simulink model "Template_TheNotebookEdition"  (R2024b)
settings: Solver=FixedStepAuto  StartTime=0.0  StopTime=inf  RelTol=1e-3  EnableMultiTasking=on
libraries: vexarmcortexlib x24, vexcommonlib x2
settings Model: Creator=ierdn  LastModifiedBy=ierdn
settings DataIOCC: LimitDataPoints=on  SignalLoggingSaveFormat=ModelDataLogs  ReturnWorkspaceOutputs=off
settings OptimizationCC: ExpressionDepthLimit=2147483647  LifeSpan=Inf  MaxStackSize=64  EfficientTunableParamExpr=on
settings DebuggingCC: UnderspecifiedInitializationDetection=Classic  MergeDetectMultiDrivingBlocksExec=none  InheritedTsInSrcMsg=none  FcnCallInpInsideContextMsg=warning  StateNameClashWarn=warning  SFUnexpectedBacktrackingDiag=warning  SFNoUnconditionalDefaultTransitionDiag=warning  SFExecutionAtInitializationDiag=none  ArithmeticOperatorsInVariantConditions=warning
settings HardwareCC: ProdBitPerPointer=32  ProdBitPerSizeT=32  ProdBitPerPtrDiffT=32  ProdLargestAtomicInteger=Long  ProdLargestAtomicFloat=Double  ProdIntDivRoundTo=Undefined  ProdWordSize=32  ProdHWDeviceType=ARM Compatible->ARM Cortex
settings ModelReferenceCC: EnableRefExpFcnMdlSchedulingChecks=on  PropagateSignalLabelsOutOfModel=off
settings SFSimCC: MATLABDynamicMemAlloc=off  CustomCodeUndefinedFunction=UseInterfaceOnly
settings RTWCC: Description=Embedded Coder  SystemTargetFile=ert.tlc  HardwareBoard=ARM Cortex-based VEX Microcontroller  TemplateMakefile=ert_default_tmf  Toolchain=GNU Tools for VEX ARM Cortex  GPUComputeCapability=3.5
settings CodeAppCC: IgnoreCustomStorageClasses=off  CustomSymbolStrType=$N$R$M  StateflowObjectComments=on  InternalIdentifier=Classic
settings ERTTargetCC: CodeReplacementLibrary=GCC ARM Cortex-M3  MultiwordLength=2048  InlinedParameterPlacement=Hierarchical  ConvertIfToSwitch=off  SuppressUnreachableDefaultCases=off  DynamicArrayContainerType=coder::array

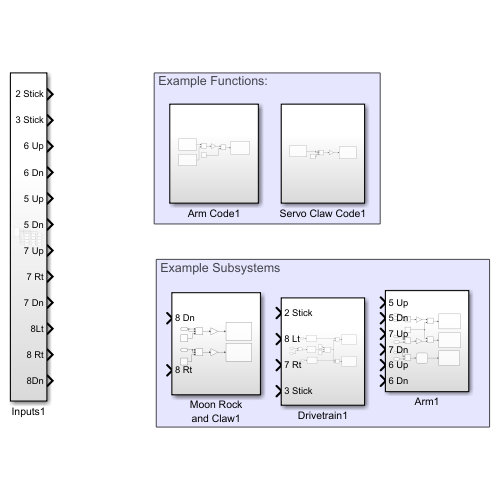
[thumbnail: Simulink's stored preview of the top-level diagram]
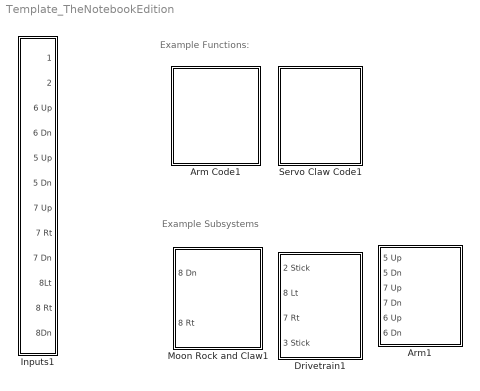
== system Template_TheNotebookEdition ==
  note: Example Functions:
  note: Example Subsystems
  Arm Code1 : Subsystem
  Arm1 : Subsystem
  Drivetrain1 : Subsystem
  Inputs1 : Subsystem
  Moon Rock and Claw1 : Subsystem
  Servo Claw Code1 : Subsystem

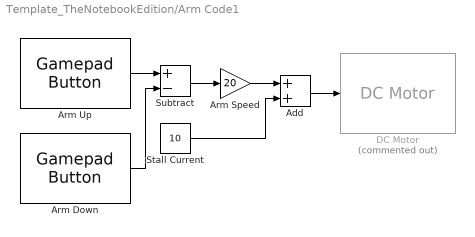
== system Template_TheNotebookEdition/Arm Code1 ==
  Add : Sum
  Arm Down : vexarmcortexlib/Gamepad/Gamepad Button  joystick=1  chan=5  button56=Down  button78=Down  SimulationIn=off  SampleTime=0.02
  Arm Speed : Gain  Gain=20
  Arm Up : vexarmcortexlib/Gamepad/Gamepad Button  joystick=1  chan=5  button56=Up  button78=Down  SimulationIn=off  SampleTime=0.02
  DC Motor : vexarmcortexlib/Actuators/DC Motor  Commented=on  motor=1  scaleFactor=1/13.5  SimulationOut=off
  Stall Current : Constant  Value=10
  Subtract : Sum  Inputs=+-
  wires:
  Arm Speed/1 -> Add/1
  Arm Down/1 -> Subtract/2
  Add/1 -> DC Motor/1
  Stall Current/1 -> Add/2
  Subtract/1 -> Arm Speed/1
  Arm Up/1 -> Subtract/1

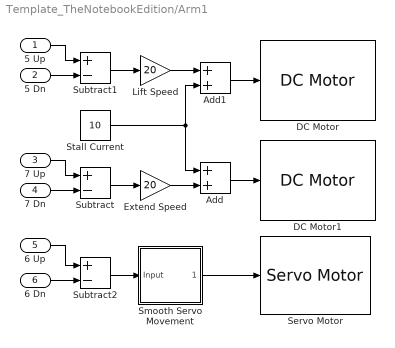
== system Template_TheNotebookEdition/Arm1 ==
  5 Up : Inport
  5 Dn : Inport  Port=2
  7 Up : Inport  Port=3
  7 Dn : Inport  Port=4
  6 Up : Inport  Port=5
  6 Dn : Inport  Port=6
  Add : Sum
  Add1 : Sum
  DC Motor : vexarmcortexlib/Actuators/DC Motor  motor=8  scaleFactor=1/13.5  SimulationOut=off
  DC Motor1 : vexarmcortexlib/Actuators/DC Motor  motor=4  scaleFactor=1/13.5  SimulationOut=off
  Extend Speed : Gain  Gain=20
  Lift Speed : Gain  Gain=20
  Servo Motor : vexarmcortexlib/Actuators/Servo Motor  motor=5  scaleFactor=60/127  SimulationOut=off
  Smooth Servo Movement : Stateflow chart  TreatAsAtomicUnit=on
  Stall Current : Constant  Value=10
  Subtract : Sum  Inputs=+-
  Subtract1 : Sum  Inputs=+-
  Subtract2 : Sum  Inputs=+-
  wires:
  5 Up/1 -> Subtract1/1
  Lift Speed/1 -> Add1/1
  Add1/1 -> DC Motor/1
  Stall Current/1 -> Add/1, Add1/2
  Subtract1/1 -> Lift Speed/1
  5 Dn/1 -> Subtract1/2
  Add/1 -> DC Motor1/1
  7 Dn/1 -> Subtract/2
  Subtract/1 -> Extend Speed/1
  Extend Speed/1 -> Add/2
  7 Up/1 -> Subtract/1
  6 Up/1 -> Subtract2/1
  6 Dn/1 -> Subtract2/2
  Subtract2/1 -> Smooth Servo Movement/1(Input)
  Smooth Servo Movement/1(Output) -> Servo Motor/1

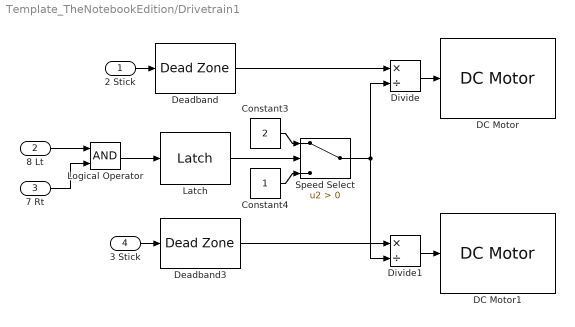
== system Template_TheNotebookEdition/Drivetrain1 ==
  2 Stick : Inport
  8 Lt : Inport  Port=2
  7 Rt : Inport  Port=3
  3 Stick : Inport  Port=4
  Constant3 : Constant  Value=2
  Constant4 : Constant
  DC Motor : vexarmcortexlib/Actuators/DC Motor  motor=2  scaleFactor=1/13.5  SimulationOut=off
  DC Motor1 : vexarmcortexlib/Actuators/DC Motor  motor=9  scaleFactor=1/13.5  SimulationOut=off
  Deadband : DeadZone  LowerValue=-9  UpperValue=9
  Deadband3 : DeadZone  LowerValue=-9  UpperValue=9
  Divide : Product  Inputs=*/
  Divide1 : Product  Inputs=*/
  Latch : vexcommonlib/Latch  output0=off  BlockPlatform=vexarmcortex
  Logical Operator : Logic  AllPortsSameDT=off  OutDataTypeStr=boolean
  Speed Select : Switch  Criteria=u2 > Threshold  SaturateOnIntegerOverflow=off  InputSameDT=off
  wires:
  Speed Select/1 -> Divide/2, Divide1/2
  Latch/1 -> Speed Select/2
  Constant3/1 -> Speed Select/1
  Deadband3/1 -> Divide1/1
  Constant4/1 -> Speed Select/3
  Deadband/1 -> Divide/1
  Divide/1 -> DC Motor/1
  3 Stick/1 -> Deadband3/1
  2 Stick/1 -> Deadband/1
  Divide1/1 -> DC Motor1/1
  8 Lt/1 -> Logical Operator/1
  7 Rt/1 -> Logical Operator/2
  Logical Operator/1 -> Latch/1

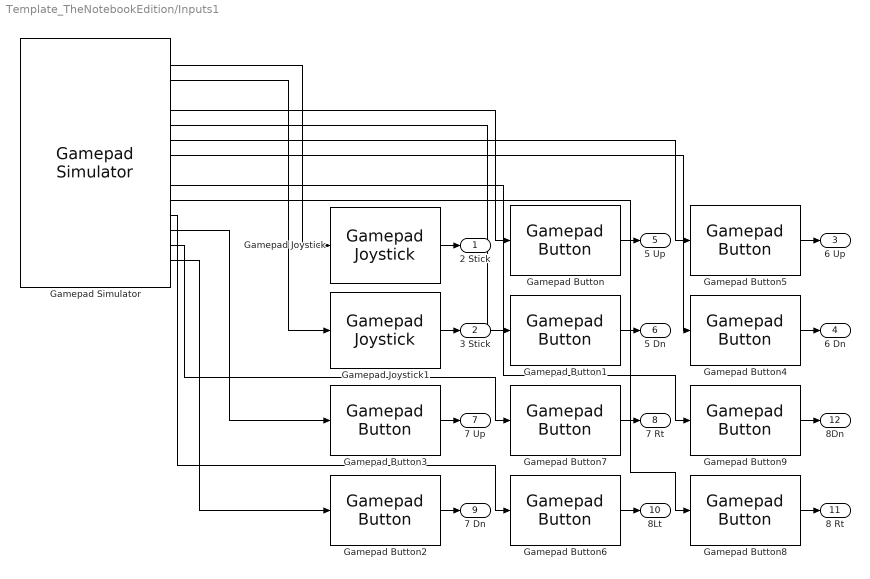
== system Template_TheNotebookEdition/Inputs1 ==
  Gamepad Button : vexarmcortexlib/Gamepad/Gamepad Button  joystick=1  chan=5  button56=Up  button78=Down  SimulationIn=on  SampleTime=0.02
  Gamepad Button1 : vexarmcortexlib/Gamepad/Gamepad Button  joystick=1  chan=5  button56=Down  button78=Down  SimulationIn=on  SampleTime=0.02
  Gamepad Button2 : vexarmcortexlib/Gamepad/Gamepad Button  joystick=1  chan=7  button56=Up  button78=Down  SimulationIn=on  SampleTime=0.02
  Gamepad Button3 : vexarmcortexlib/Gamepad/Gamepad Button  joystick=1  chan=7  button56=Up  button78=Up  SimulationIn=on  SampleTime=0.02
  Gamepad Button4 : vexarmcortexlib/Gamepad/Gamepad Button  joystick=1  chan=6  button56=Down  button78=Down  SimulationIn=on  SampleTime=0.02
  Gamepad Button5 : vexarmcortexlib/Gamepad/Gamepad Button  joystick=1  chan=6  button56=Up  button78=Down  SimulationIn=on  SampleTime=0.02
  Gamepad Button6 : vexarmcortexlib/Gamepad/Gamepad Button  joystick=1  chan=8  button56=Up  button78=Left  SimulationIn=on  SampleTime=0.02
  Gamepad Button7 : vexarmcortexlib/Gamepad/Gamepad Button  joystick=1  chan=7  button56=Up  button78=Right  SimulationIn=on  SampleTime=0.02
  Gamepad Button8 : vexarmcortexlib/Gamepad/Gamepad Button  joystick=1  chan=8  button56=Up  button78=Right  SimulationIn=on  SampleTime=0.02
  Gamepad Button9 : vexarmcortexlib/Gamepad/Gamepad Button  joystick=1  chan=8  button56=Up  button78=Down  SimulationIn=on  SampleTime=0.02
  Gamepad Joystick : vexarmcortexlib/Gamepad/Gamepad Joystick  joystick=1  chan=2  SimulationIn=on  SampleTime=0.02
  Gamepad Joystick1 : vexarmcortexlib/Gamepad/Gamepad Joystick  joystick=1  chan=3  SimulationIn=on  SampleTime=0.02
  Gamepad Simulator : vexcommonlib/Gamepad Simulator  WhichPad=Logitech Gamepad  JoyId=1  BlockPlatform=vexarmcortex
      settings: LibrarySourceBlock=vexarmcortexlib/Utilities/Gamepad Simulator
  " 2 Stick" : Outport
  3 Stick : Outport  Port=2
  6 Up : Outport  Port=3
  6 Dn : Outport  Port=4
  5 Up : Outport  Port=5
  5 Dn : Outport  Port=6
  7 Up : Outport  Port=7
  7 Rt : Outport  Port=8
  7 Dn : Outport  Port=9
  8Lt : Outport  Port=10
  8 Rt : Outport  Port=11
  8Dn : Outport  Port=12
  wires:
  Gamepad Button5/1 -> 6 Up/1
  Gamepad Joystick1/1 -> 3 Stick/1
  Gamepad Button9/1 -> 8Dn/1
  Gamepad Button6/1 -> 8Lt/1
  Gamepad Button7/1 -> 7 Rt/1
  Gamepad Button4/1 -> 6 Dn/1
  Gamepad Button1/1 -> 5 Dn/1
  Gamepad Button/1 -> 5 Up/1
  Gamepad Button8/1 -> 8 Rt/1
  Gamepad Button3/1 -> 7 Up/1
  Gamepad Button2/1 -> 7 Dn/1
  Gamepad Joystick/1 -> " 2 Stick"/1
  Gamepad Simulator/2 -> Gamepad Joystick/1
  Gamepad Simulator/3 -> Gamepad Joystick1/1
  Gamepad Simulator/13 -> Gamepad Button3/1
  Gamepad Simulator/15 -> Gamepad Button2/1
  Gamepad Simulator/14 -> Gamepad Button7/1
  Gamepad Simulator/12 -> Gamepad Button6/1
  Gamepad Simulator/5 -> Gamepad Button/1
  Gamepad Simulator/6 -> Gamepad Button1/1
  Gamepad Simulator/7 -> Gamepad Button5/1
  Gamepad Simulator/8 -> Gamepad Button4/1
  Gamepad Simulator/10 -> Gamepad Button9/1
  Gamepad Simulator/11 -> Gamepad Button8/1

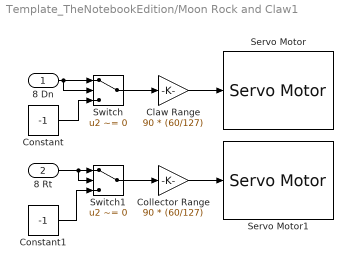
== system Template_TheNotebookEdition/Moon Rock and Claw1 ==
  8 Dn : Inport
  8 Rt : Inport  Port=2
  Claw Range : Gain  Gain=90 * (60/127)
  Collector Range : Gain  Gain=90 * (60/127)
  Constant : Constant  Value=-1
  Constant1 : Constant  Value=-1
  Servo Motor : vexarmcortexlib/Actuators/Servo Motor  motor=6  scaleFactor=60/127  SimulationOut=off
  Servo Motor1 : vexarmcortexlib/Actuators/Servo Motor  motor=7  scaleFactor=60/127  SimulationOut=off
  Switch : Switch  Criteria=u2 ~= 0  SaturateOnIntegerOverflow=off  InputSameDT=off
  Switch1 : Switch  Criteria=u2 ~= 0  SaturateOnIntegerOverflow=off  InputSameDT=off
  wires:
  Switch1/1 -> Collector Range/1
  8 Dn/1 -> Switch/2, Switch/1
  8 Rt/1 -> Switch1/2, Switch1/1
  Collector Range/1 -> Servo Motor1/1
  Constant1/1 -> Switch1/3
  Claw Range/1 -> Servo Motor/1
  Switch/1 -> Claw Range/1
  Constant/1 -> Switch/3

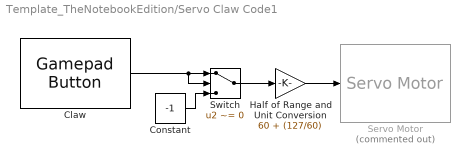
== system Template_TheNotebookEdition/Servo Claw Code1 ==
  Claw : vexarmcortexlib/Gamepad/Gamepad Button  joystick=1  chan=7  button56=Up  button78=Down  SimulationIn=off  SampleTime=0.02
  Constant : Constant  Value=-1
  Half of Range and Unit Conversion : Gain  Gain=60 + (127/60)
  Servo Motor : vexarmcortexlib/Actuators/Servo Motor  Commented=on  motor=1  scaleFactor=60/127  SimulationOut=off
  Switch : Switch  Criteria=u2 ~= 0  SaturateOnIntegerOverflow=off  InputSameDT=off
  wires:
  Claw/1 -> Switch/2, Switch/1
  Switch/1 -> Half of Range and Unit Conversion/1
  Constant/1 -> Switch/3
  Half of Range and Unit Conversion/1 -> Servo Motor/1

== stateflow chart Template_TheNotebookEdition/Arm1/Smooth Servo Movement ==
  state Constant
    Speed = 0.5;
  state Change
    Output=Output+(Input*Speed);
  (default) -> Constant : {Output = 0}
  Constant -> Change : [(Input ~= 0)&&(Output >= -127 || Input == 1)&&(Output <= 127 || Input == -1)]
  Change -> Constant
  data: Input input; Output output; Speed local
